simulink model "DRIPDemo001"  (Simulink 8.3)
settings: Solver=ode45  StartTime=0.0  StopTime=10.0  RelTol=1e-3
model workspace (MAT data in the model file):
  MPS_Models = {'..\..\..\solutions\demos\models\demos\Demo001.mps'}
  variantInfo = VariabilitySupport
  variantInfo.name = 'CityVariabilityModel1'
  variantInfo.featureModels(1) = FeatureModel
  variantInfo.featureModels(1).id = 'pmCa98Oxt$'
  variantInfo.featureModels(1).name = 'desktopOrHIL'
  variantInfo.featureModels(1).root = Feature
  variantInfo.featureModels(1).root.id = 'pmCa98Oxt_'
  variantInfo.featureModels(1).root.children(1) = Feature
  variantInfo.featureModels(1).root.children(1).id = 'pmCa98Oxw_'
  variantInfo.featureModels(1).root.children(1).name = 'MIL'
  variantInfo.featureModels(1).root.children(2) = Feature
  variantInfo.featureModels(1).root.children(2).id = 'pmCa98OxwD'
  variantInfo.featureModels(1).root.children(2).name = 'HIL'
  variantInfo.featureModels(2) = FeatureModel
  variantInfo.featureModels(2).id = '4psHK0ldtYc'
  variantInfo.featureModels(2).name = 'creep_mode'
  variantInfo.featureModels(2).root = Feature
  variantInfo.featureModels(2).root.id = '4psHK0ldtYd'
  variantInfo.featureModels(2).root.children(1) = Feature
  variantInfo.featureModels(2).root.children(1).id = '63tTPuP4CV9'
  variantInfo.featureModels(2).root.children(1).name = 'creeptype'
  variantInfo.featureModels(2).root.children(1).children(1) = Feature
  variantInfo.featureModels(2).root.children(1).children(1).id = '63tTPuP4CVe'
  variantInfo.featureModels(2).root.children(1).children(1).name = 'highCreep'
  variantInfo.featureModels(2).root.children(1).children(2) = Feature
  variantInfo.featureModels(2).root.children(1).children(2).id = '63tTPuP4CVh'
  variantInfo.featureModels(2).root.children(1).children(2).name = 'lowCreep'
  variantInfo.featureModels(2).root.children(2) = Feature
  variantInfo.featureModels(2).root.children(2).id = '63tTPuP4CVo'
  variantInfo.featureModels(2).root.children(2).name = 'region'
  variantInfo.featureModels(2).root.children(2).children(1) = Feature
  variantInfo.featureModels(2).root.children(2).children(1).id = '63tTPuP4CVv'
  variantInfo.featureModels(2).root.children(2).children(1).name = 'Asia'
  variantInfo.featureModels(2).root.children(2).children(2) = Feature
  variantInfo.featureModels(2).root.children(2).children(2).id = '63tTPuP4CVy'
  variantInfo.featureModels(2).root.children(2).children(2).name = 'US'
  variantInfo.featureModels(3) = FeatureModel
  variantInfo.featureModels(3).id = '57MGTm6KTqG'
  variantInfo.featureModels(3).name = 'IAC_ETC'
  variantInfo.featureModels(3).root = Feature
  variantInfo.featureModels(3).root.id = '57MGTm6KTqH'
  variantInfo.featureModels(3).root.children(1) = Feature
  variantInfo.featureModels(3).root.children(1).id = '57MGTm6KTrb'
  variantInfo.featureModels(3).root.children(1).name = 'IAC'
  variantInfo.featureModels(3).root.children(1).children(1) = Feature
  variantInfo.featureModels(3).root.children(1).children(1).id = '57MGTm6KTrk'
  variantInfo.featureModels(3).root.children(1).children(1).name = 'WithIAC'
  variantInfo.featureModels(3).root.children(1).children(2) = Feature
  variantInfo.featureModels(3).root.children(1).children(2).id = '57MGTm6KTr_'
  variantInfo.featureModels(3).root.children(1).children(2).name = 'WithoutIAC'
  variantInfo.featureModels(3).root.children(2) = Feature
  variantInfo.featureModels(3).root.children(2).id = '57MGTm6KTrd'
  variantInfo.featureModels(3).root.children(2).name = 'ETC'
  variantInfo.featureModels(3).root.children(2).children(1) = Feature
  variantInfo.featureModels(3).root.children(2).children(1).id = '57MGTm6KTrD'
  variantInfo.featureModels(3).root.children(2).children(1).name = 'WithETC'
  variantInfo.featureModels(3).root.children(2).children(2) = Feature
  variantInfo.featureModels(3).root.children(2).children(2).id = '57MGTm6KTrG'
  variantInfo.featureModels(3).root.children(2).children(2).name = 'ManualThrottle'
  variantInfo.featureModels(4) = FeatureModel
  variantInfo.featureModels(4).id = '5nH12nXhsEk'
  variantInfo.featureModels(4).name = 'PTArch'
  variantInfo.featureModels(4).root = Feature
  variantInfo.featureModels(4).root.id = '5nH12nXhsEl'
  variantInfo.featureModels(4).root.children(1) = Feature
  variantInfo.featureModels(4).root.children(1).id = '5nH12nXhsGF'
  variantInfo.featureModels(4).root.children(1).name = 'lumped'
  variantInfo.featureModels(4).root.children(2) = Feature
  variantInfo.featureModels(4).root.children(2).id = '5nH12nXhsGS'
  variantInfo.featureModels(4).root.children(2).name = 'separate'
  variantInfo.configModels(1) = VariantConfigurationModel
  variantInfo.configModels(1).id = 'pmCa98Ox$4'
  variantInfo.configModels(1).name = 'MILsim'
  variantInfo.configModels(1).featureRef = MpsObjectRef
  variantInfo.configModels(1).featureRef.targetNodeId = 'pmCa98Oxt$'
  variantInfo.configModels(1).featureRef.resolveInfo = 'desktopOrHIL'
  variantInfo.configModels(1).rootFeature = VariantSelectedFeature
  variantInfo.configModels(1).rootFeature.featureRef = MpsObjectRef
  variantInfo.configModels(1).rootFeature.featureRef.targetNodeId = 'pmCa98Oxt_'
  variantInfo.configModels(1).rootFeature.featureRef.resolveInfo = 'desktopOrHIL_root'
  variantInfo.configModels(1).rootFeature.children = VariantSelectedFeature
  variantInfo.configModels(1).rootFeature.children.featureRef = MpsObjectRef
  variantInfo.configModels(1).rootFeature.children.featureRef.targetNodeId = 'pmCa98Oxw_'
  variantInfo.configModels(1).rootFeature.children.featureRef.resolveInfo = 'MIL'
  variantInfo.configModels(2) = VariantConfigurationModel
  variantInfo.configModels(2).id = 'pmCa98OxEI'
  variantInfo.configModels(2).name = 'HILsim'
  variantInfo.configModels(2).featureRef = MpsObjectRef
  variantInfo.configModels(2).featureRef.targetNodeId = 'pmCa98Oxt$'
  variantInfo.configModels(2).featureRef.resolveInfo = 'desktopOrHIL'
  variantInfo.configModels(2).rootFeature = VariantSelectedFeature
  variantInfo.configModels(2).rootFeature.featureRef = MpsObjectRef
  variantInfo.configModels(2).rootFeature.featureRef.targetNodeId = 'pmCa98Oxt_'
  variantInfo.configModels(2).rootFeature.featureRef.resolveInfo = 'desktopOrHIL_root'
  variantInfo.configModels(2).rootFeature.children = VariantSelectedFeature
  variantInfo.configModels(2).rootFeature.children.featureRef = MpsObjectRef
  variantInfo.configModels(2).rootFeature.children.featureRef.targetNodeId = 'pmCa98OxwD'
  variantInfo.configModels(2).rootFeature.children.featureRef.resolveInfo = 'HIL'
  variantInfo.configModels(3) = VariantConfigurationModel
  variantInfo.configModels(3).id = '4psHK0ldtYh'
  variantInfo.configModels(3).name = 'HighCreepJP'
  variantInfo.configModels(3).featureRef = MpsObjectRef
  variantInfo.configModels(3).featureRef.targetNodeId = '4psHK0ldtYc'
  variantInfo.configModels(3).featureRef.resolveInfo = 'creep_mode'
  variantInfo.configModels(3).rootFeature = VariantSelectedFeature
  variantInfo.configModels(3).rootFeature.featureRef = MpsObjectRef
  variantInfo.configModels(3).rootFeature.featureRef.targetNodeId = '4psHK0ldtYd'
  variantInfo.configModels(3).rootFeature.featureRef.resolveInfo = 'creep_mode_root'
  variantInfo.configModels(3).rootFeature.children(1) = VariantSelectedFeature
  variantInfo.configModels(3).rootFeature.children(1).featureRef = MpsObjectRef
  variantInfo.configModels(3).rootFeature.children(1).featureRef.targetNodeId = '63tTPuP4CV9'
  variantInfo.configModels(3).rootFeature.children(1).featureRef.resolveInfo = 'creeptype'
  variantInfo.configModels(3).rootFeature.children(1).children = VariantSelectedFeature
  variantInfo.configModels(3).rootFeature.children(1).children.featureRef = MpsObjectRef
  variantInfo.configModels(3).rootFeature.children(1).children.featureRef.targetNodeId = '63tTPuP4CVe'
  variantInfo.configModels(3).rootFeature.children(1).children.featureRef.resolveInfo = 'highCreep'
  variantInfo.configModels(3).rootFeature.children(2) = VariantSelectedFeature
  variantInfo.configModels(3).rootFeature.children(2).featureRef = MpsObjectRef
  variantInfo.configModels(3).rootFeature.children(2).featureRef.targetNodeId = '63tTPuP4CVo'
  variantInfo.configModels(3).rootFeature.children(2).featureRef.resolveInfo = 'region'
  variantInfo.configModels(3).rootFeature.children(2).children = VariantSelectedFeature
  variantInfo.configModels(3).rootFeature.children(2).children.featureRef = MpsObjectRef
  variantInfo.configModels(3).rootFeature.children(2).children.featureRef.targetNodeId = '63tTPuP4CVv'
  variantInfo.configModels(3).rootFeature.children(2).children.featureRef.resolveInfo = 'Asia'
  variantInfo.configModels(4) = VariantConfigurationModel
  variantInfo.configModels(4).id = '4psHK0ldtYk'
  variantInfo.configModels(4).name = 'LowCreepUS'
  variantInfo.configModels(4).featureRef = MpsObjectRef
  variantInfo.configModels(4).featureRef.targetNodeId = '4psHK0ldtYc'
  variantInfo.configModels(4).featureRef.resolveInfo = 'creep_mode'
  variantInfo.configModels(4).rootFeature = VariantSelectedFeature
  variantInfo.configModels(4).rootFeature.featureRef = MpsObjectRef
  variantInfo.configModels(4).rootFeature.featureRef.targetNodeId = '4psHK0ldtYd'
  variantInfo.configModels(4).rootFeature.featureRef.resolveInfo = 'creep_mode_root'
  variantInfo.configModels(4).rootFeature.children(1) = VariantSelectedFeature
  variantInfo.configModels(4).rootFeature.children(1).featureRef = MpsObjectRef
  variantInfo.configModels(4).rootFeature.children(1).featureRef.targetNodeId = '63tTPuP4CV9'
  variantInfo.configModels(4).rootFeature.children(1).featureRef.resolveInfo = 'creeptype'
  variantInfo.configModels(4).rootFeature.children(1).children = VariantSelectedFeature
  variantInfo.configModels(4).rootFeature.children(1).children.featureRef = MpsObjectRef
  variantInfo.configModels(4).rootFeature.children(1).children.featureRef.targetNodeId = '63tTPuP4CVh'
  variantInfo.configModels(4).rootFeature.children(1).children.featureRef.resolveInfo = 'lowCreep'
  variantInfo.configModels(4).rootFeature.children(2) = VariantSelectedFeature
  variantInfo.configModels(4).rootFeature.children(2).featureRef = MpsObjectRef
  variantInfo.configModels(4).rootFeature.children(2).featureRef.targetNodeId = '63tTPuP4CVo'
  variantInfo.configModels(4).rootFeature.children(2).featureRef.resolveInfo = 'region'
  variantInfo.configModels(4).rootFeature.children(2).children = VariantSelectedFeature
  variantInfo.configModels(4).rootFeature.children(2).children.featureRef = MpsObjectRef
  variantInfo.configModels(4).rootFeature.children(2).children.featureRef.targetNodeId = '63tTPuP4CVy'
  variantInfo.configModels(4).rootFeature.children(2).children.featureRef.resolveInfo = 'US'
  variantInfo.configModels(5) = VariantConfigurationModel
  variantInfo.configModels(5).id = '57MGTm6KTsn'
  variantInfo.configModels(5).name = 'ManualThrottle'
  variantInfo.configModels(5).featureRef = MpsObjectRef
  variantInfo.configModels(5).featureRef.targetNodeId = '57MGTm6KTqG'
  variantInfo.configModels(5).featureRef.resolveInfo = 'IAC_ETC'
  variantInfo.configModels(5).rootFeature = VariantSelectedFeature
  variantInfo.configModels(5).rootFeature.featureRef = MpsObjectRef
  variantInfo.configModels(5).rootFeature.featureRef.targetNodeId = '57MGTm6KTqH'
  variantInfo.configModels(5).rootFeature.featureRef.resolveInfo = 'IAC_ETC_root'
  variantInfo.configModels(5).rootFeature.children(1) = VariantSelectedFeature
  variantInfo.configModels(5).rootFeature.children(1).featureRef = MpsObjectRef
  variantInfo.configModels(5).rootFeature.children(1).featureRef.targetNodeId = '57MGTm6KTrb'
  variantInfo.configModels(5).rootFeature.children(1).featureRef.resolveInfo = 'IAC'
  variantInfo.configModels(5).rootFeature.children(1).children = VariantSelectedFeature
  variantInfo.configModels(5).rootFeature.children(1).children.featureRef = MpsObjectRef
  variantInfo.configModels(5).rootFeature.children(1).children.featureRef.targetNodeId = '57MGTm6KTrk'
  variantInfo.configModels(5).rootFeature.children(1).children.featureRef.resolveInfo = 'WithIAC'
  variantInfo.configModels(5).rootFeature.children(2) = VariantSelectedFeature
  variantInfo.configModels(5).rootFeature.children(2).featureRef = MpsObjectRef
  variantInfo.configModels(5).rootFeature.children(2).featureRef.targetNodeId = '57MGTm6KTrd'
  variantInfo.configModels(5).rootFeature.children(2).featureRef.resolveInfo = 'ETC'
  variantInfo.configModels(5).rootFeature.children(2).children = VariantSelectedFeature
  variantInfo.configModels(5).rootFeature.children(2).children.featureRef = MpsObjectRef
  variantInfo.configModels(5).rootFeature.children(2).children.featureRef.targetNodeId = '57MGTm6KTrG'
  variantInfo.configModels(5).rootFeature.children(2).children.featureRef.resolveInfo = 'ManualThrottle'
  variantInfo.configModels(6) = VariantConfigurationModel
  variantInfo.configModels(6).id = '57MGTm6KTu4'
  variantInfo.configModels(6).name = 'HybridETC'
  variantInfo.configModels(6).featureRef = MpsObjectRef
  variantInfo.configModels(6).featureRef.targetNodeId = '57MGTm6KTqG'
  variantInfo.configModels(6).featureRef.resolveInfo = 'IAC_ETC'
  variantInfo.configModels(6).rootFeature = VariantSelectedFeature
  variantInfo.configModels(6).rootFeature.featureRef = MpsObjectRef
  variantInfo.configModels(6).rootFeature.featureRef.targetNodeId = '57MGTm6KTqH'
  variantInfo.configModels(6).rootFeature.featureRef.resolveInfo = 'IAC_ETC_root'
  variantInfo.configModels(6).rootFeature.children(1) = VariantSelectedFeature
  variantInfo.configModels(6).rootFeature.children(1).featureRef = MpsObjectRef
  variantInfo.configModels(6).rootFeature.children(1).featureRef.targetNodeId = '57MGTm6KTrb'
  variantInfo.configModels(6).rootFeature.children(1).featureRef.resolveInfo = 'IAC'
  variantInfo.configModels(6).rootFeature.children(1).children = VariantSelectedFeature
  variantInfo.configModels(6).rootFeature.children(1).children.featureRef = MpsObjectRef
  variantInfo.configModels(6).rootFeature.children(1).children.featureRef.targetNodeId = '57MGTm6KTrk'
  variantInfo.configModels(6).rootFeature.children(1).children.featureRef.resolveInfo = 'WithIAC'
  variantInfo.configModels(6).rootFeature.children(2) = VariantSelectedFeature
  variantInfo.configModels(6).rootFeature.children(2).featureRef = MpsObjectRef
  variantInfo.configModels(6).rootFeature.children(2).featureRef.targetNodeId = '57MGTm6KTrd'
  variantInfo.configModels(6).rootFeature.children(2).featureRef.resolveInfo = 'ETC'
  variantInfo.configModels(6).rootFeature.children(2).children = VariantSelectedFeature
  variantInfo.configModels(6).rootFeature.children(2).children.featureRef = MpsObjectRef
  variantInfo.configModels(6).rootFeature.children(2).children.featureRef.targetNodeId = '57MGTm6KTrD'
  variantInfo.configModels(6).rootFeature.children(2).children.featureRef.resolveInfo = 'WithETC'
  variantInfo.configModels(7) = VariantConfigurationModel
  variantInfo.configModels(7).id = '57MGTm6KTvT'
  variantInfo.configModels(7).name = 'RegularETC'
  variantInfo.configModels(7).featureRef = MpsObjectRef
  variantInfo.configModels(7).featureRef.targetNodeId = '57MGTm6KTqG'
  variantInfo.configModels(7).featureRef.resolveInfo = 'IAC_ETC'
  variantInfo.configModels(7).rootFeature = VariantSelectedFeature
  variantInfo.configModels(7).rootFeature.featureRef = MpsObjectRef
  variantInfo.configModels(7).rootFeature.featureRef.targetNodeId = '57MGTm6KTqH'
  variantInfo.configModels(7).rootFeature.featureRef.resolveInfo = 'IAC_ETC_root'
  variantInfo.configModels(7).rootFeature.children(1) = VariantSelectedFeature
  variantInfo.configModels(7).rootFeature.children(1).featureRef = MpsObjectRef
  variantInfo.configModels(7).rootFeature.children(1).featureRef.targetNodeId = '57MGTm6KTrb'
  variantInfo.configModels(7).rootFeature.children(1).featureRef.resolveInfo = 'IAC'
  variantInfo.configModels(7).rootFeature.children(1).children = VariantSelectedFeature
  variantInfo.configModels(7).rootFeature.children(1).children.featureRef = MpsObjectRef
  variantInfo.configModels(7).rootFeature.children(1).children.featureRef.targetNodeId = '57MGTm6KTr_'
  variantInfo.configModels(7).rootFeature.children(1).children.featureRef.resolveInfo = 'WithoutIAC'
  variantInfo.configModels(7).rootFeature.children(2) = VariantSelectedFeature
  variantInfo.configModels(7).rootFeature.children(2).featureRef = MpsObjectRef
  variantInfo.configModels(7).rootFeature.children(2).featureRef.targetNodeId = '57MGTm6KTrd'
  variantInfo.configModels(7).rootFeature.children(2).featureRef.resolveInfo = 'ETC'
  variantInfo.configModels(7).rootFeature.children(2).children = VariantSelectedFeature
  variantInfo.configModels(7).rootFeature.children(2).children.featureRef = MpsObjectRef
  variantInfo.configModels(7).rootFeature.children(2).children.featureRef.targetNodeId = '57MGTm6KTrD'
  variantInfo.configModels(7).rootFeature.children(2).children.featureRef.resolveInfo = 'WithETC'
  MPS_ModuleName = 'DEMOS.Demo001'
PostLoadFcn:
  | loadDRIReqsInfo('DRIPDemo001', []);
PreSaveFcn:
  | modelWS=get_param('DRIPDemo001', 'modelworkspace');modelWS.evalin('clear driModuleInfo simModuleInfo');clear modelWS;
settings Model: Creator=swami  LastModifiedBy=swami
settings DataIOCC: SignalLoggingSaveFormat=Dataset
settings DebuggingCC: UnderspecifiedInitializationDetection=Simplified  StateNameClashWarn=none
settings GRTTargetCC: CombineOutputUpdateFcns=on  GRTInterface=off

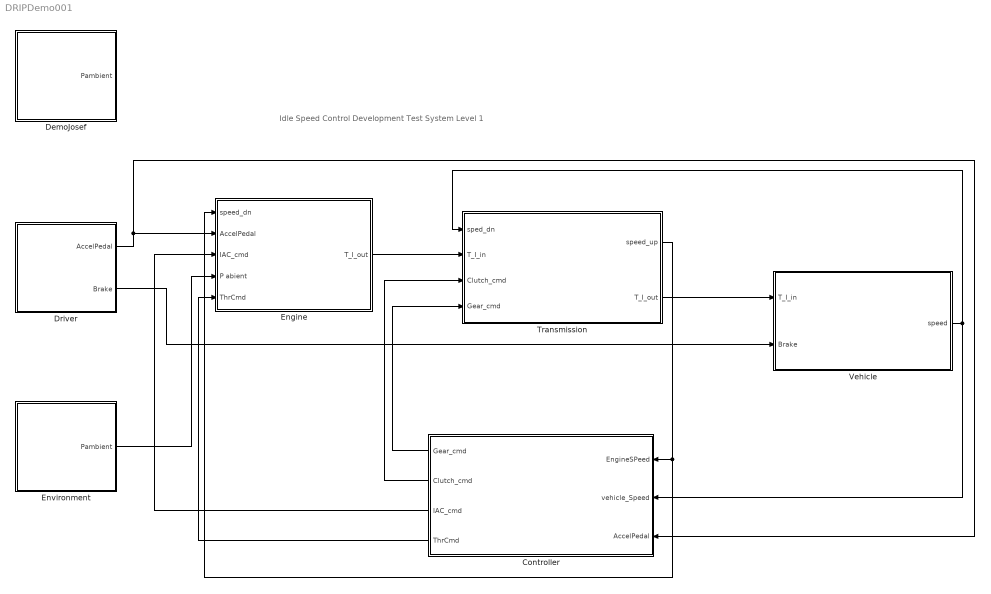
== system DRIPDemo001 ==
  note: Idle Speed Control Development Test System
      | Level 1
  Controller : Subsystem
  DemoJosef : Subsystem
  Driver : Subsystem
  Engine : Subsystem
  Environment : Subsystem
  Transmission : Subsystem
  Vehicle : Subsystem
  wires:
  Driver/1(AccelPedal) -> Controller/3(AccelPedal), Engine/2(AccelPedal)
  Engine/1(T_I_out) -> Transmission/2(T_I_in)
  Transmission/1(speed_up) -> Engine/1(speed_dn), Controller/1(EngineSPeed)
  Transmission/2(T_I_out) -> Vehicle/1(T_I_in)
  Driver/2(Brake) -> Vehicle/2(Brake)
  Vehicle/1(speed) -> Controller/2(vehicle_Speed), Transmission/1(sped_dn)
  Controller/1(Gear_cmd) -> Transmission/4(Gear_cmd)
  Controller/2(Clutch_cmd) -> Transmission/3(Clutch_cmd)
  Controller/3(IAC_cmd) -> Engine/3(IAC_cmd)
  Environment/1(Pambient) -> Engine/4(P abient)
  Controller/4(ThrCmd) -> Engine/5(ThrCmd)

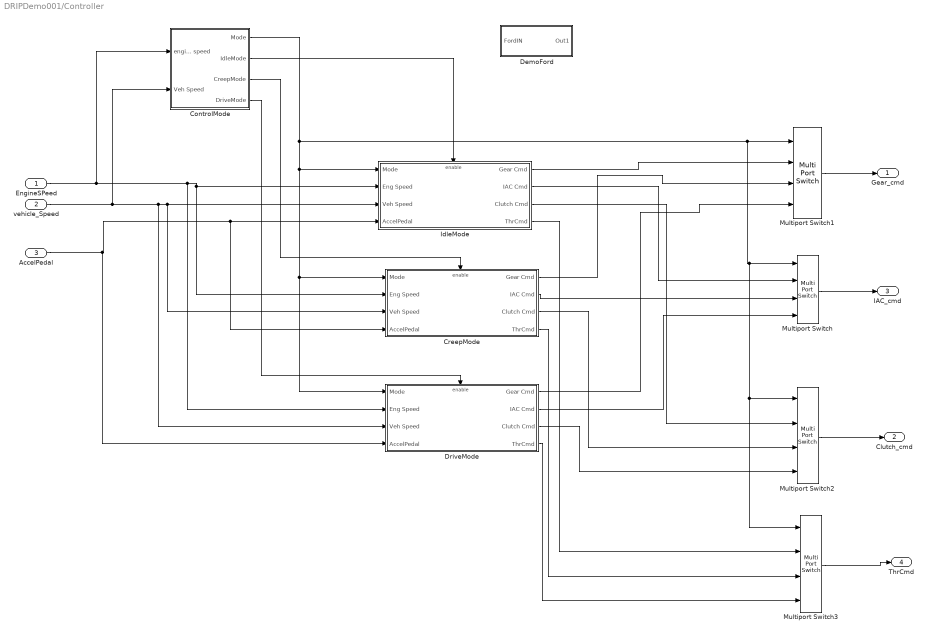
== system DRIPDemo001/Controller ==
  EngineSPeed : Inport
  vehicle_Speed : Inport  Port=2
  AccelPedal : Inport  Port=3
  ControlMode : Subsystem
  CreepMode : Subsystem
  DemoFord : Subsystem
  DriveMode : Subsystem
  IdleMode : Subsystem
  Multiport Switch{,1..3} (4 alike) : MultiPortSwitch
  Gear_cmd : Outport
  Clutch_cmd : Outport  Port=2
  IAC_cmd : Outport  Port=3
  ThrCmd : Outport  Port=4
  wires:
  ControlMode/1(Mode) -> Multiport Switch3/1, Multiport Switch2/1, Multiport Switch/1, Multiport Switch1/1, DriveMode/1(Mode), CreepMode/1(Mode), IdleMode/1(Mode)
  ControlMode/2(IdleMode) -> IdleMode/Enable
  ControlMode/3(CreepMode) -> CreepMode/Enable
  ControlMode/4(DriveMode) -> DriveMode/Enable
  EngineSPeed/1 -> ControlMode/1(engine speed), DriveMode/2(Eng Speed), CreepMode/2(Eng Speed), IdleMode/2(Eng Speed)
  vehicle_Speed/1 -> ControlMode/2(Veh Speed), DriveMode/3(Veh Speed), CreepMode/3(Veh Speed), IdleMode/3(Veh Speed)
  IdleMode/1(Gear Cmd) -> Multiport Switch1/2
  CreepMode/1(Gear Cmd) -> Multiport Switch1/3
  DriveMode/1(Gear Cmd) -> Multiport Switch1/4
  Multiport Switch1/1 -> Gear_cmd/1
  IdleMode/2(IAC Cmd) -> Multiport Switch/2
  CreepMode/2(IAC Cmd) -> Multiport Switch/3
  DriveMode/2(IAC Cmd) -> Multiport Switch/4
  Multiport Switch/1 -> IAC_cmd/1
  IdleMode/3(Clutch Cmd) -> Multiport Switch2/2
  CreepMode/3(Clutch Cmd) -> Multiport Switch2/3
  DriveMode/3(Clutch Cmd) -> Multiport Switch2/4
  Multiport Switch2/1 -> Clutch_cmd/1
  Multiport Switch3/1 -> ThrCmd/1
  IdleMode/4(ThrCmd) -> Multiport Switch3/2
  CreepMode/4(ThrCmd) -> Multiport Switch3/3
  DriveMode/4(ThrCmd) -> Multiport Switch3/4
  AccelPedal/1 -> DriveMode/4(AccelPedal), CreepMode/4(AccelPedal), IdleMode/4(AccelPedal)

== system DRIPDemo001/DemoJosef ==
  Pambient : Outport

== system DRIPDemo001/Driver ==
  AccelPedal : Outport
  Brake : Outport  Port=2
  wires:
  ? -> Brake/1

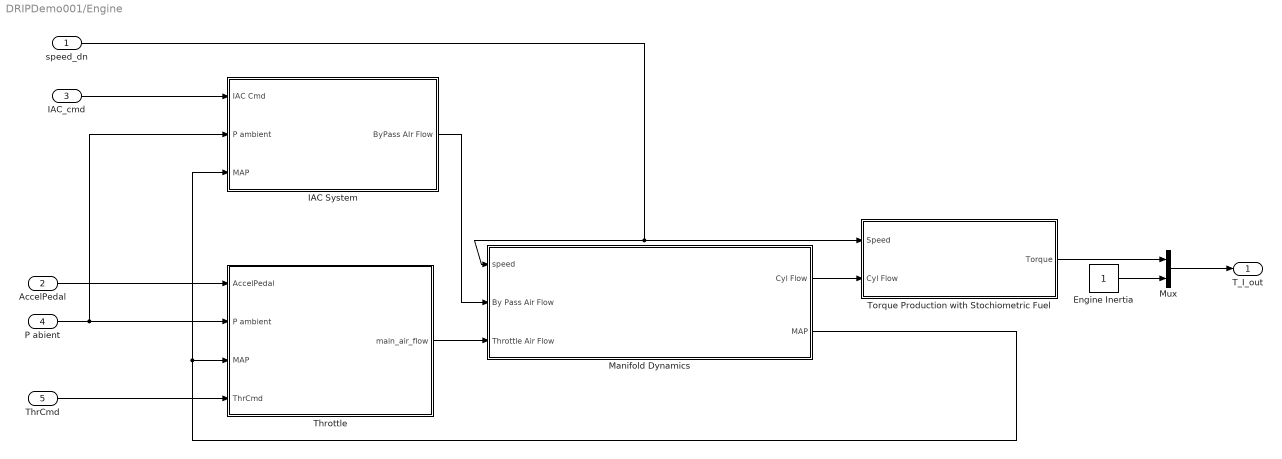
== system DRIPDemo001/Engine ==
  speed_dn : Inport
  AccelPedal : Inport  Port=2
  IAC_cmd : Inport  Port=3
  P abient : Inport  Port=4
  ThrCmd : Inport  Port=5
  Engine Inertia : Constant
  IAC System : Subsystem  Variant=on  OverrideUsingVariant=Variant4
  Manifold Dynamics : Subsystem
  Mux : Mux  Inputs=2
  Throttle : Subsystem  Variant=on  OverrideUsingVariant=Variant3
  Torque Production with Stochiometric Fuel : Subsystem
  T_I_out : Outport
  wires:
  Manifold Dynamics/2(MAP) -> IAC System/3(MAP), Throttle/3(MAP)
  P abient/1 -> IAC System/2(P ambient), Throttle/2(P ambient)
  AccelPedal/1 -> Throttle/1(AccelPedal)
  IAC_cmd/1 -> IAC System/1(IAC Cmd)
  IAC System/1(ByPass AIr Flow) -> Manifold Dynamics/2(By Pass Air Flow)
  Throttle/1(main_air_flow) -> Manifold Dynamics/3(Throttle Air Flow)
  speed_dn/1 -> Torque Production with Stochiometric Fuel/1(Speed), Manifold Dynamics/1(speed)
  Manifold Dynamics/1(Cyl Flow) -> Torque Production with Stochiometric Fuel/2(Cyl Flow)
  Engine Inertia/1 -> Mux/2
  Torque Production with Stochiometric Fuel/1(Torque) -> Mux/1
  Mux/1 -> T_I_out/1
  ThrCmd/1 -> Throttle/4(ThrCmd)

== system DRIPDemo001/Environment ==
  Pambient : Outport

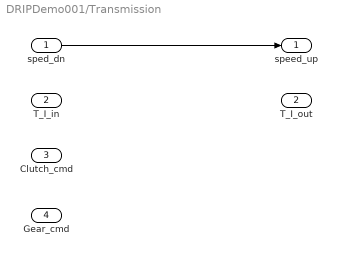
== system DRIPDemo001/Transmission ==
  sped_dn : Inport
  T_I_in : Inport  Port=2
  Clutch_cmd : Inport  Port=3
  Gear_cmd : Inport  Port=4
  speed_up : Outport
  T_I_out : Outport  Port=2
  wires:
  sped_dn/1 -> speed_up/1

== system DRIPDemo001/Vehicle ==
  T_I_in : Inport
  Brake : Inport  Port=2
  speed : Outport
  wires:
  T_I_in/1 -> speed/1

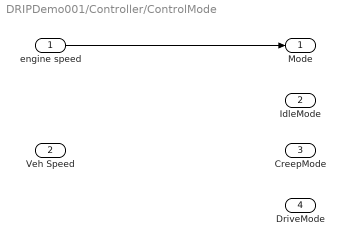
== system DRIPDemo001/Controller/ControlMode ==
  engine speed : Inport
  Veh Speed : Inport  Port=2
  Mode : Outport
  IdleMode : Outport  Port=2
  CreepMode : Outport  Port=3
  DriveMode : Outport  Port=4
  wires:
  engine speed/1 -> Mode/1

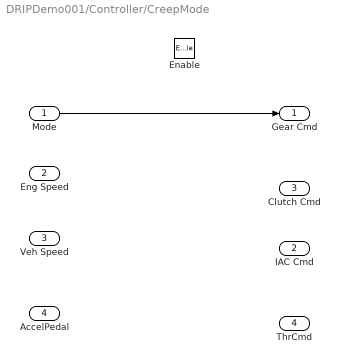
== system DRIPDemo001/Controller/CreepMode ==
  Mode : Inport
  Eng Speed : Inport  Port=2
  Veh Speed : Inport  Port=3
  AccelPedal : Inport  Port=4
  Enable : EnablePort
  Gear Cmd : Outport
  IAC Cmd : Outport  Port=2
  Clutch Cmd : Outport  Port=3
  ThrCmd : Outport  Port=4
  wires:
  Mode/1 -> Gear Cmd/1

== system DRIPDemo001/Controller/DemoFord ==
  FordIN : Inport
  Out1 : Outport
  wires:
  FordIN/1 -> Out1/1

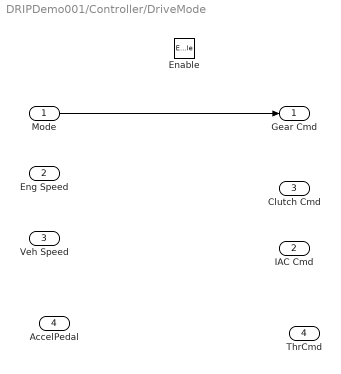
== system DRIPDemo001/Controller/DriveMode ==
  Mode : Inport
  Eng Speed : Inport  Port=2
  Veh Speed : Inport  Port=3
  AccelPedal : Inport  Port=4
  Enable : EnablePort
  Gear Cmd : Outport
  IAC Cmd : Outport  Port=2
  Clutch Cmd : Outport  Port=3
  ThrCmd : Outport  Port=4
  wires:
  Mode/1 -> Gear Cmd/1

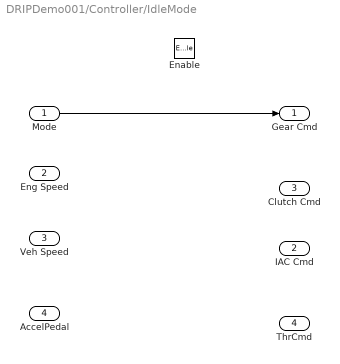
== system DRIPDemo001/Controller/IdleMode ==
  Mode : Inport
  Eng Speed : Inport  Port=2
  Veh Speed : Inport  Port=3
  AccelPedal : Inport  Port=4
  Enable : EnablePort
  Gear Cmd : Outport
  IAC Cmd : Outport  Port=2
  Clutch Cmd : Outport  Port=3
  ThrCmd : Outport  Port=4
  wires:
  Mode/1 -> Gear Cmd/1

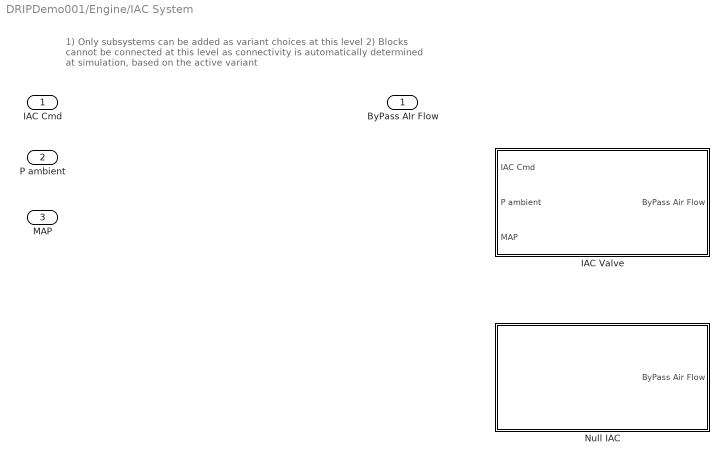
== system DRIPDemo001/Engine/IAC System ==
  note: 1) Only subsystems can be added as variant choices at this level
      | 2) Blocks cannot be connected at this level as connectivity is
      | automatically determined at simulation, based on the active variant
  IAC Cmd : Inport
  P ambient : Inport  Port=2
  MAP : Inport  Port=3
  IAC Valve : Subsystem  VariantControl=Variant3
  Null IAC : Subsystem  VariantControl=Variant4
  ByPass AIr Flow : Outport

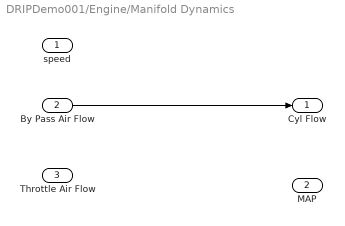
== system DRIPDemo001/Engine/Manifold Dynamics ==
  speed : Inport
  By Pass Air Flow : Inport  Port=2
  Throttle Air Flow : Inport  Port=3
  Cyl Flow : Outport
  MAP : Outport  Port=2
  wires:
  By Pass Air Flow/1 -> Cyl Flow/1

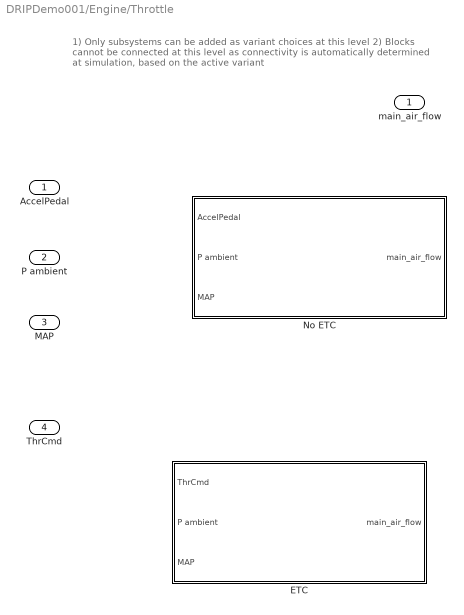
== system DRIPDemo001/Engine/Throttle ==
  note: 1) Only subsystems can be added as variant choices at this level
      | 2) Blocks cannot be connected at this level as connectivity is
      | automatically determined at simulation, based on the active variant
  AccelPedal : Inport
  P ambient : Inport  Port=2
  MAP : Inport  Port=3
  ThrCmd : Inport  Port=4
  ETC : Subsystem  VariantControl=Variant3
  No ETC : Subsystem  VariantControl=Variant4
  main_air_flow : Outport

== system DRIPDemo001/Engine/Torque Production with Stochiometric Fuel ==
  Speed : Inport
  Cyl Flow : Inport  Port=2
  Torque : Outport
  wires:
  Cyl Flow/1 -> Torque/1

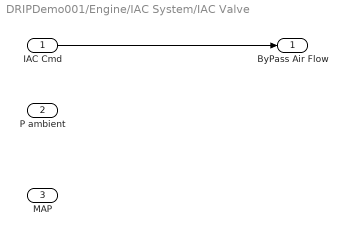
== system DRIPDemo001/Engine/IAC System/IAC Valve ==
  IAC Cmd : Inport
  P ambient : Inport  Port=2
  MAP : Inport  Port=3
  ByPass Air Flow : Outport
  wires:
  IAC Cmd/1 -> ByPass Air Flow/1

== system DRIPDemo001/Engine/IAC System/Null IAC ==
  zero : Constant  Value=0
  ByPass Air Flow : Outport
  wires:
  zero/1 -> ByPass Air Flow/1

== system DRIPDemo001/Engine/Throttle/ETC ==
  ThrCmd : Inport
  P ambient : Inport  Port=2
  MAP : Inport  Port=3
  main_air_flow : Outport
  wires:
  ThrCmd/1 -> main_air_flow/1

== system DRIPDemo001/Engine/Throttle/No ETC ==
  AccelPedal : Inport
  P ambient : Inport  Port=2
  MAP : Inport  Port=3
  main_air_flow : Outport
  wires:
  AccelPedal/1 -> main_air_flow/1
